simulink model "HPP_Shell_18"  (R2018a)
settings: Solver=VariableStepAuto  StartTime=0.0  StopTime=10.0  RelTol=1e-3
settings Model: Creator=Sohan  LastModifiedBy=Sohan

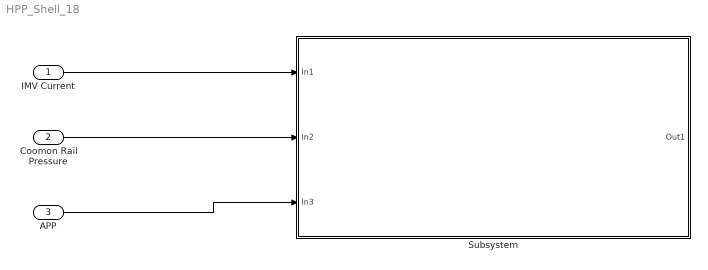
== system HPP_Shell_18 ==
  IMV Current : Inport
  Coomon Rail Pressure : Inport  Port=2
  APP : Inport  Port=3
  Subsystem : Subsystem
  wires:
  IMV Current/1 -> Subsystem/1(In1)
  Coomon Rail Pressure/1 -> Subsystem/2(In2)
  APP/1 -> Subsystem/3(In3)

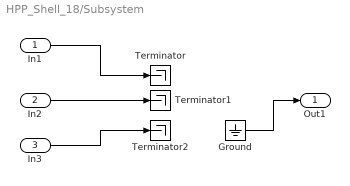
== system HPP_Shell_18/Subsystem ==
  In1 : Inport
  In2 : Inport  Port=2
  In3 : Inport  Port=3
  Ground : Ground
  Terminator : Terminator
  Terminator1 : Terminator
  Terminator2 : Terminator
  Out1 : Outport
  wires:
  In3/1 -> Terminator2/1
  In2/1 -> Terminator1/1
  In1/1 -> Terminator/1
  Ground/1 -> Out1/1
